simulink model "kalmanov_regulator"  (R2018a)
settings: Solver=ode4  StartTime=0.0  StopTime=500  FixedStep=0.01  RelTol=1e-3  EnableMultiTasking=on
values from neighbouring files (symbols this model uses):
  Ak = [df1_H1 df1_H2 df1_theta_m; df2_H1 df2_H2 df2_theta_m; df3_H1 df3_H2 df3_theta_m]    [skript_prvi_deo.m]
  Bk = [df1_Uvh df1_Uvt df1_Uv2; df2_Uvh df2_Uvt df2_Uv2; df3_Uvh df3_Uvt df3_Uv2]    [skript_prvi_deo.m]
  Ck = [1 0 0; 0 1 0; 0 0 1]    [skript_prvi_deo.m]
  Dk = [0 0 0; 0 0 0; 0 0 0]    [skript_prvi_deo.m]
  K = K    [skript_prvi_deo.m]
settings Model: Creator=Nikola  LastModifiedBy=lakim
settings DataIOCC: LimitDataPoints=on  SaveFormat=Array
settings OptimizationCC: LifeSpan=inf
settings DebuggingCC: SFUnexpectedBacktrackingDiag=warning  SFNoUnconditionalDefaultTransitionDiag=warning  SFExecutionAtInitializationDiag=none
settings HardwareCC: ProdBitPerPointer=32  ProdBitPerSizeT=32  ProdBitPerPtrDiffT=32  ProdLargestAtomicFloat=None  ProdIntDivRoundTo=Undefined  ProdEndianess=Unspecified  ProdWordSize=32  ProdHWDeviceType=32-bit Generic
settings ModelReferenceCC: PropagateSignalLabelsOutOfModel=off
settings CodeAppCC: StateflowObjectComments=on
settings GRTTargetCC: TargetLangStandard=C89/C90 (ANSI)  GeneratePreprocessorConditionals=Disable all
settings ConfigComp: CovMetricSettings=dw  CovHtmlReporting=on  CovSaveCumulativeToWorkspaceVar=on  CovSaveSingleToWorkspaceVar=on  CovExternalEMLEnable=off

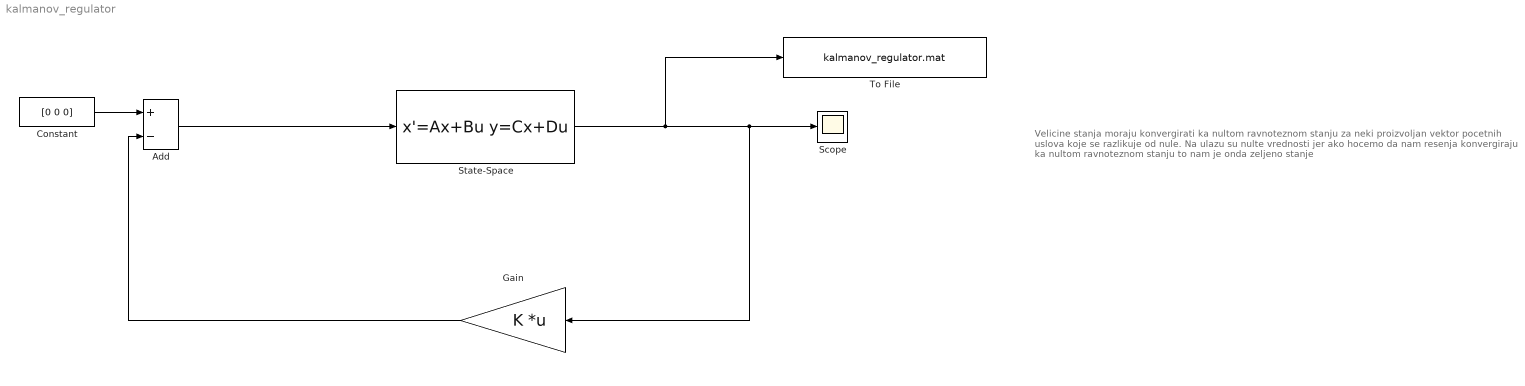
== system kalmanov_regulator ==
  note: Velicine stanja moraju konvergirati ka nultom ravnoteznom stanju za neki proizvoljan vektor pocetnih uslova koje se razlikuje od nule. Na ulazu su nulte vrednosti jer ako hocemo da nam resenja konvergiraju ka nultom ravnoteznom stanju to nam je onda zeljeno stanje
  Add : Sum  Inputs=+-
  Constant : Constant  Value=[0 0 0]
  Gain : Gain  Gain=K  Multiplication=Matrix(K*u)
  Scope : Scope
  State-Space : StateSpace  A=Ak  B=Bk  C=Ck  D=Dk  InitialCondition=[2 3 4]
  To File : ToFile  Filename=kalmanov_regulator.mat  MatrixName=k
  wires:
  State-Space/1 -> To File/1, Scope/1, Gain/1
  Gain/1 -> Add/2
  Constant/1 -> Add/1
  Add/1 -> State-Space/1
